simulink model "H13"  (Simulink 7.3)
settings: Solver=ode45  StartTime=0.0  StopTime=4  RelTol=1e-3
libraries: simulink x1
settings Model: Creator=Sainquake  LastModifiedBy=Sainquake

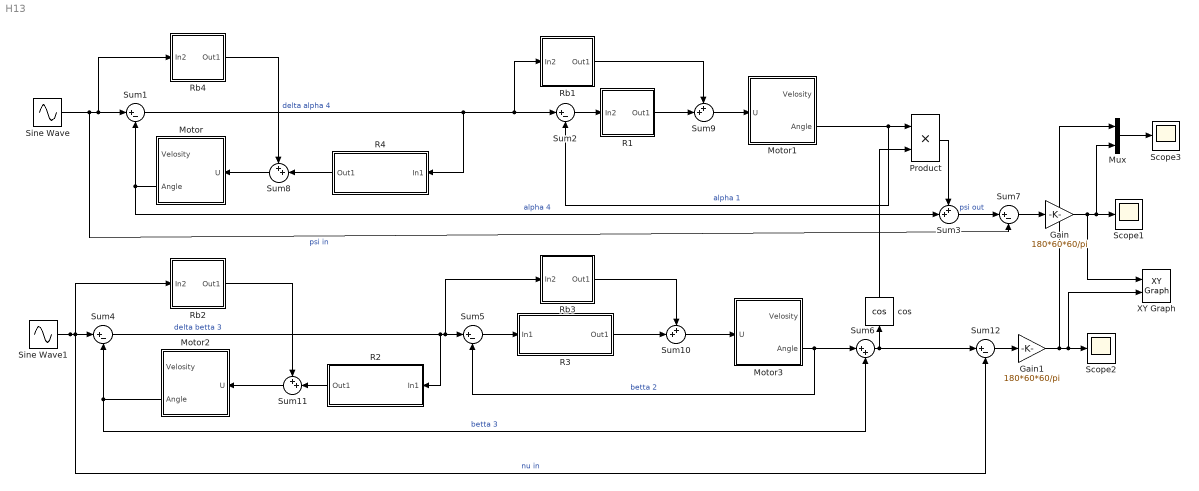
== system H13 ==
  Gain : Gain  Gain=180*60*60/pi  ParameterDataType=fixdt(1, 16)  ParameterScaling=2^0  OutDataType=fixdt(1, 16)  OutScaling=2^0
  Gain1 : Gain  Gain=180*60*60/pi  ParameterDataType=fixdt(1, 16)  ParameterScaling=2^0  OutDataType=fixdt(1, 16)  OutScaling=2^0
  Motor : Subsystem  TreatAsAtomicUnit=on
  Motor1 : Subsystem  TreatAsAtomicUnit=on
  Motor2 : Subsystem  TreatAsAtomicUnit=on
  Motor3 : Subsystem  TreatAsAtomicUnit=on
  Mux : Mux  Inputs=2
  Product : Product  OutDataType=fixdt(1, 16)  OutScaling=2^0  RndMeth=Zero
  R1 : Subsystem
  R2 : Subsystem
  R3 : Subsystem
  R4 : Subsystem
  Rb1 : Subsystem
  Rb2 : Subsystem
  Rb3 : Subsystem
  Rb4 : Subsystem
  Scope1 : Scope
      settings: YMin=-1250  YMax=1500  MaxDataPoints=500000
  Scope2 : Scope
      settings: MaxDataPoints=500000
  Scope3 : Scope
      settings: YMin=-1250  YMax=1500  SaveName=ScopeData2  MaxDataPoints=500000
  Sine Wave : Sin  Amplitude=1  Bias=0  Frequency=1  Phase=0  Samples=10  SampleTime=0  Offset=0
  Sine Wave1 : Sin  Amplitude=1  Bias=0  Frequency=1  Phase=0  Samples=10  SampleTime=0  Offset=0
  Sum{1..2,4..5,7,12} (6 alike) : Sum  Inputs=|+-  OutDataType=fixdt(1, 16)  OutScaling=2^0
  Sum{3,8..11} (5 alike) : Sum  Inputs=++|  OutDataType=fixdt(1, 16)  OutScaling=2^0
  Sum6 : Sum  Inputs=|++  OutDataType=fixdt(1, 16)  OutScaling=2^0
  XY Graph : simulink/Sinks/XY Graph  SystemSampleTime=-1  xmin=-3*1280  xmax=3*1280  ymin=-3*960  ymax=3*960  st=-1
  cos : Trigonometry  Operator=cos
  wires:
  R4/1(Out1) -> Sum8/2
  Motor1/2(Angle) -> Product/1, Sum2/2  "alpha 1"
  Sum2/1 -> R1/1(In2)
  Product/1 -> Sum3/1
  Sum3/1 -> Sum7/1  "psi out"
  Motor/2(Angle) -> Sum1/2, Sum3/2  "alpha 4"
  R2/1(Out1) -> Sum11/2
  Sum4/1 -> R2/1(In1), Sum5/1, Rb3/1(In2)  "delta betta 3"
  Sine Wave1/1 -> Sum4/1, Rb2/1(In2), Sum12/2  "nu in"
  R3/1(Out1) -> Sum10/2
  Motor3/2(Angle) -> Sum5/2, Sum6/1  "betta 2"
  Sum5/1 -> R3/1(In1)
  Motor2/2(Angle) -> Sum4/2, Sum6/2  "betta 3"
  Sum6/1 -> cos/1, Sum12/1
  Sine Wave/1 -> Sum1/1, Rb4/1(In2), Sum7/2  "psi in"
  Rb1/1(Out1) -> Sum9/1
  Rb4/1(Out1) -> Sum8/1
  R1/1(Out1) -> Sum9/2
  Sum9/1 -> Motor1/1(U)
  Sum8/1 -> Motor/1(U)
  Rb2/1(Out1) -> Sum11/1
  Sum11/1 -> Motor2/1(U)
  Sum10/1 -> Motor3/1(U)
  Rb3/1(Out1) -> Sum10/1
  Sum7/1 -> Gain/1
  Gain/1 -> XY Graph/1, Scope1/1, Mux/2
  Sum1/1 -> Sum2/1, Rb1/1(In2), R4/1(In1)  "delta alpha 4"
  Gain1/1 -> Scope2/1, XY Graph/2, Mux/1
  Sum12/1 -> Gain1/1
  cos/1 -> Product/2
  Mux/1 -> Scope3/1

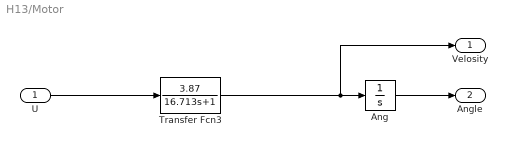
== system H13/Motor ==
  U : Inport  OutDataType=fixdt(1, 16)  OutScaling=2^0
  Ang : Integrator
  Transfer Fcn3 : TransferFcn  Numerator=[3.87]  Denominator=[16.713 1]
  Velosity : Outport  OutDataType=fixdt(1, 16)  OutScaling=2^0
  Angle : Outport  Port=2  OutDataType=fixdt(1, 16)  OutScaling=2^0
  wires:
  Ang/1 -> Angle/1
  U/1 -> Transfer Fcn3/1
  Transfer Fcn3/1 -> Ang/1, Velosity/1

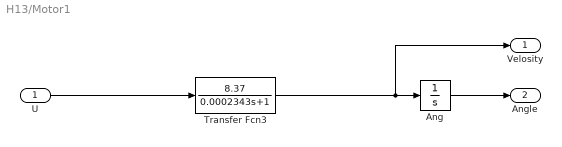
== system H13/Motor1 ==
  U : Inport  OutDataType=fixdt(1, 16)  OutScaling=2^0
  Ang : Integrator
  Transfer Fcn3 : TransferFcn  Numerator=[8.37]  Denominator=[0.0002343 1]
  Velosity : Outport  OutDataType=fixdt(1, 16)  OutScaling=2^0
  Angle : Outport  Port=2  OutDataType=fixdt(1, 16)  OutScaling=2^0
  wires:
  Ang/1 -> Angle/1
  U/1 -> Transfer Fcn3/1
  Transfer Fcn3/1 -> Ang/1, Velosity/1

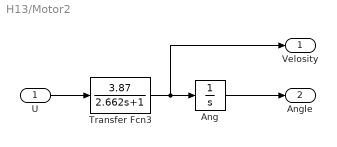
== system H13/Motor2 ==
  U : Inport  OutDataType=fixdt(1, 16)  OutScaling=2^0
  Ang : Integrator
  Transfer Fcn3 : TransferFcn  Numerator=[3.87]  Denominator=[2.662 1]
  Velosity : Outport  OutDataType=fixdt(1, 16)  OutScaling=2^0
  Angle : Outport  Port=2  OutDataType=fixdt(1, 16)  OutScaling=2^0
  wires:
  Ang/1 -> Angle/1
  U/1 -> Transfer Fcn3/1
  Transfer Fcn3/1 -> Ang/1, Velosity/1

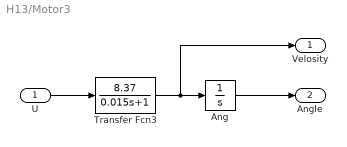
== system H13/Motor3 ==
  U : Inport  OutDataType=fixdt(1, 16)  OutScaling=2^0
  Ang : Integrator
  Transfer Fcn3 : TransferFcn  Numerator=[8.37]  Denominator=[0.015 1]
  Velosity : Outport  OutDataType=fixdt(1, 16)  OutScaling=2^0
  Angle : Outport  Port=2  OutDataType=fixdt(1, 16)  OutScaling=2^0
  wires:
  Ang/1 -> Angle/1
  U/1 -> Transfer Fcn3/1
  Transfer Fcn3/1 -> Ang/1, Velosity/1

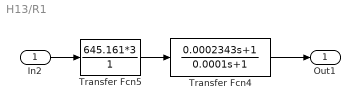
== system H13/R1 ==
  In2 : Inport  OutDataType=fixdt(1, 16)  OutScaling=2^0
  Transfer Fcn4 : TransferFcn  Numerator=[0.0002343 1]  Denominator=[0.0001 1]
  Transfer Fcn5 : TransferFcn  Numerator=645.161*3  Denominator=1
  Out1 : Outport  OutDataType=fixdt(1, 16)  OutScaling=2^0
  wires:
  Transfer Fcn5/1 -> Transfer Fcn4/1
  Transfer Fcn4/1 -> Out1/1
  In2/1 -> Transfer Fcn5/1

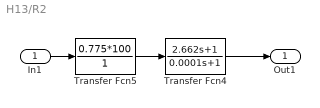
== system H13/R2 ==
  In1 : Inport  OutDataType=fixdt(1, 16)  OutScaling=2^0
  Transfer Fcn4 : TransferFcn  Numerator=[2.662 1]  Denominator=[0.0001 1]
  Transfer Fcn5 : TransferFcn  Numerator=0.775*100  Denominator=1
  Out1 : Outport  OutDataType=fixdt(1, 16)  OutScaling=2^0
  wires:
  In1/1 -> Transfer Fcn5/1
  Transfer Fcn5/1 -> Transfer Fcn4/1
  Transfer Fcn4/1 -> Out1/1

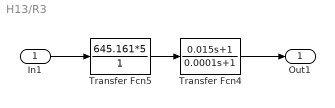
== system H13/R3 ==
  In1 : Inport  OutDataType=fixdt(1, 16)  OutScaling=2^0
  Transfer Fcn4 : TransferFcn  Numerator=[0.015 1]  Denominator=[0.0001 1]
  Transfer Fcn5 : TransferFcn  Numerator=645.161*5  Denominator=1
  Out1 : Outport  OutDataType=fixdt(1, 16)  OutScaling=2^0
  wires:
  In1/1 -> Transfer Fcn5/1
  Transfer Fcn5/1 -> Transfer Fcn4/1
  Transfer Fcn4/1 -> Out1/1

== system H13/R4 ==
  In1 : Inport  OutDataType=fixdt(1, 16)  OutScaling=2^0
  Transfer Fcn1 : TransferFcn  Numerator=[16.713 1]  Denominator=[0.0001 1]
  Transfer Fcn2 : TransferFcn  Numerator=0.775*100  Denominator=1
  Out1 : Outport  OutDataType=fixdt(1, 16)  OutScaling=2^0
  wires:
  In1/1 -> Transfer Fcn2/1
  Transfer Fcn1/1 -> Out1/1
  Transfer Fcn2/1 -> Transfer Fcn1/1

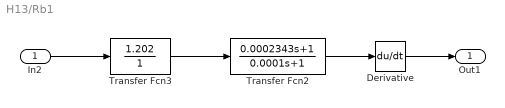
== system H13/Rb1 ==
  In2 : Inport  OutDataType=fixdt(1, 16)  OutScaling=2^0
  Derivative : Derivative
  Transfer Fcn2 : TransferFcn  Numerator=[0.0002343 1]  Denominator=[0.0001 1]
  Transfer Fcn3 : TransferFcn  Numerator=1.202  Denominator=1
  Out1 : Outport  OutDataType=fixdt(1, 16)  OutScaling=2^0
  wires:
  Derivative/1 -> Out1/1
  Transfer Fcn2/1 -> Derivative/1
  Transfer Fcn3/1 -> Transfer Fcn2/1
  In2/1 -> Transfer Fcn3/1

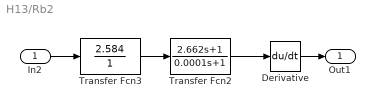
== system H13/Rb2 ==
  In2 : Inport  OutDataType=fixdt(1, 16)  OutScaling=2^0
  Derivative : Derivative
  Transfer Fcn2 : TransferFcn  Numerator=[2.662 1]  Denominator=[0.0001 1]
  Transfer Fcn3 : TransferFcn  Numerator=2.584  Denominator=1
  Out1 : Outport  OutDataType=fixdt(1, 16)  OutScaling=2^0
  wires:
  Transfer Fcn3/1 -> Transfer Fcn2/1
  Transfer Fcn2/1 -> Derivative/1
  Derivative/1 -> Out1/1
  In2/1 -> Transfer Fcn3/1

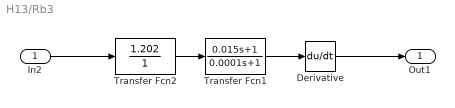
== system H13/Rb3 ==
  In2 : Inport  OutDataType=fixdt(1, 16)  OutScaling=2^0
  Derivative : Derivative
  Transfer Fcn1 : TransferFcn  Numerator=[0.015 1]  Denominator=[0.0001 1]
  Transfer Fcn2 : TransferFcn  Numerator=1.202  Denominator=1
  Out1 : Outport  OutDataType=fixdt(1, 16)  OutScaling=2^0
  wires:
  In2/1 -> Transfer Fcn2/1
  Derivative/1 -> Out1/1
  Transfer Fcn2/1 -> Transfer Fcn1/1
  Transfer Fcn1/1 -> Derivative/1

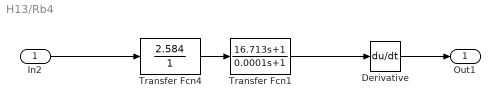
== system H13/Rb4 ==
  In2 : Inport  OutDataType=fixdt(1, 16)  OutScaling=2^0
  Derivative : Derivative
  Transfer Fcn1 : TransferFcn  Numerator=[16.713 1]  Denominator=[0.0001 1]
  Transfer Fcn4 : TransferFcn  Numerator=2.584  Denominator=1
  Out1 : Outport  OutDataType=fixdt(1, 16)  OutScaling=2^0
  wires:
  Derivative/1 -> Out1/1
  Transfer Fcn1/1 -> Derivative/1
  In2/1 -> Transfer Fcn4/1
  Transfer Fcn4/1 -> Transfer Fcn1/1
